simulink model "compositeload"  (R2023b)
settings: Solver=ode23t  StartTime=0.0  StopTime=30  RelTol=1e-2
libraries: spsThreePhaseDynamicLoadLib x3, spsAsynchronousMachinepuUnitsLib x3, spsThreePhaseVIMeasurementLib x3, spsThreePhaseSeriesRLCLoadLib x2, spsPower3phPhasorLib x1, spsThreePhasePISectionLineLib x1, spsThreePhaseTransformerTwoWindingsLib x1, spsThreePhaseBreakerLib x1, spsThreePhaseFaultLib x1, spsThreePhaseSourceLib x1, sps_lib x1
settings Model: Creator=Md. Kibria Saroare  LastModifiedBy=Md. Kibria Saroare

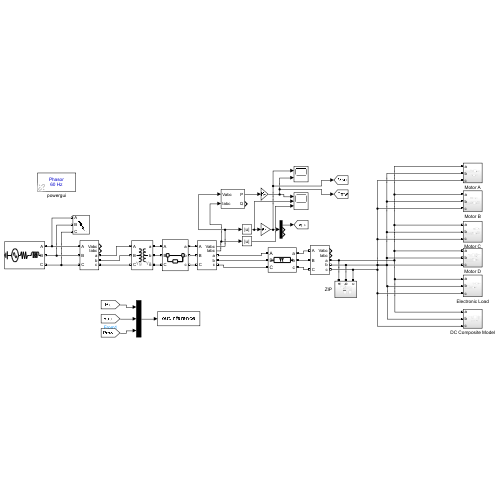
[thumbnail: Simulink's stored preview of the top-level diagram]
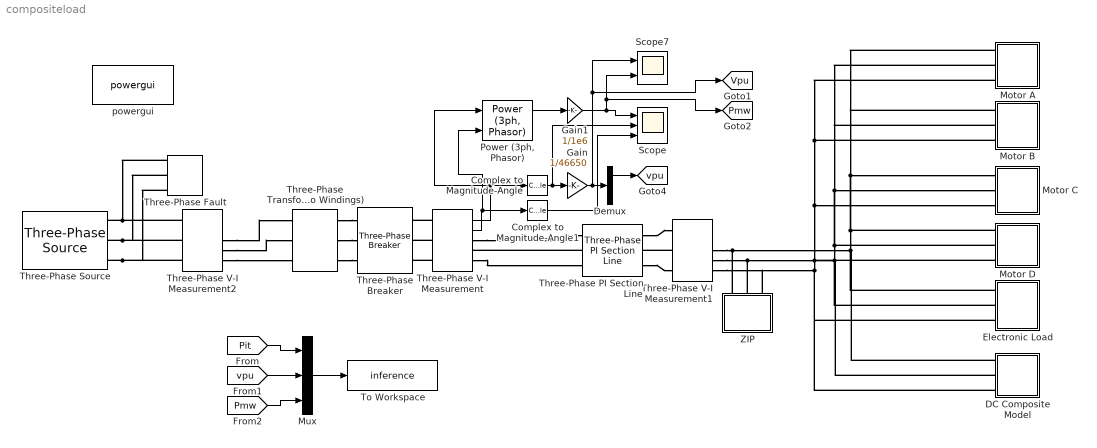
== system compositeload ==
  Complex to Magnitude-Angle : ComplexToMagnitudeAngle  Output=Magnitude
  Complex to Magnitude-Angle1 : ComplexToMagnitudeAngle  Output=Magnitude
  DC Composite Model : Subsystem
  Demux : Demux  Outputs=3
  Electronic Load : Subsystem
  Gain : Gain  Gain=1/46650
  Gain1 : Gain  Gain=1/1e6
  Motor A : Subsystem
  Motor B : Subsystem
  Motor C : Subsystem
  Motor D : Subsystem
  Mux : Mux  Inputs=3
  "Power (3ph, Phasor)" : spsPower3phPhasorLib/Power (3ph, Phasor)
      settings: LibrarySourceBlock=|
      | sps_lib/Sensors and Measurements/Power
      | (3ph, Phasor)
  Scope : Scope  NumInputPorts=3
  Scope7 : Scope  NumInputPorts=2
  Three-Phase PI Section Line : spsThreePhasePISectionLineLib/Three-Phase PI Section Line  LConnTagsString=a|b|c  RConnTagsString=A|B|C  Length=1  Frequency=60  Resistances=[ 0.3485 1.0455]  Inductances="[ 9.243e-4  2.773e-3]"  Capacitances=[1e-6 1e-6]
  Three-Phase Transformer (Two Windings) : spsThreePhaseTransformerTwoWindingsLib/Three-Phase Transformer (Two Windings)  Winding1Connection=Yg  Winding2Connection=Yg  CoreType=Three single-phase transformers  SetSaturation=off  Hysteresis=off  DataFile='hysteresis'  SetInitialFlux=off  Measurements=None  UNITS=pu  NominalPower=[ 2000e6 , 60 ]  Winding1=[2.3e+05 0.005 0.04]  Winding2=[33000 0.005 0.04]  Rm=500  Lm=500  L0=0.5  Saturation=[0 0;0.00035329 0.13044;0.1472 0.16522]  InitialFluxes=[ 0.8 , -0.8 , 0.7 ]  BreakLoop=off  DiscreteSolver=Trapezoidal iterative  DataType=off  TransfoNumber=1
  Three-Phase V-I Measurement : spsThreePhaseVIMeasurementLib/Three-Phase V-I Measurement  VoltageMeasurement=phase-to-phase  SetLabelV=off  LabelV=Vabc  Vpu=off  VpuLL=off  CurrentMeasurement=yes  SetLabelI=off  LabelI=Iabc  Ipu=off  Pbase=100e6  Vbase=500e3  OutputType=Complex  PhasorSimulation=on  PSBequivalent=0
  Three-Phase V-I Measurement1 : spsThreePhaseVIMeasurementLib/Three-Phase V-I Measurement  VoltageMeasurement=phase-to-phase  SetLabelV=off  LabelV=Vabc  Vpu=off  VpuLL=off  CurrentMeasurement=yes  SetLabelI=off  LabelI=Iabc  Ipu=off  Pbase=100e6  Vbase=500e3  OutputType=Complex  PhasorSimulation=on  PSBequivalent=0
  Three-Phase V-I Measurement2 : spsThreePhaseVIMeasurementLib/Three-Phase V-I Measurement  VoltageMeasurement=phase-to-phase  SetLabelV=off  LabelV=Vabc  Vpu=off  VpuLL=off  CurrentMeasurement=yes  SetLabelI=off  LabelI=Iabc  Ipu=off  Pbase=100e6  Vbase=500e3  OutputType=Complex  PhasorSimulation=on  PSBequivalent=0
  Three-Phase Breaker : spsThreePhaseBreakerLib/Three-Phase Breaker  InitialState=closed  SwitchA=on  SwitchB=on  SwitchC=on  SwitchTimes="[1/60  5/60]"  External=off  BreakerResistance=0.0001  SnubberResistance=1e6  SnubberCapacitance=inf  Measurements=None
  Three-Phase Fault : spsThreePhaseFaultLib/Three-Phase Fault  InitialStates=0  FaultA=on  FaultB=on  FaultC=on  GroundFault=on  SwitchTimes="[4  4.6]"  External=off  SwitchStatus=NaN  FaultResistance=0.001  GroundResistance=0.01  SnubberResistance=1e6  SnubberCapacitance=inf  Measurements=None
  Three-Phase Source : spsThreePhaseSourceLib/Three-Phase Source  InternalConnection=Yg  VoltagePhases=off  Voltage=230e3  PhaseAngle=0  Voltage_phases=[25e3 25e3 25e3]/sqrt(3)  PhaseAngles_phases=[0 -120 +120]  Frequency=60  NonIdealSource=on  SpecifyImpedance=on  Resistance=0.8929  Inductance=16.58e-3  ShortCircuitLevel=20000e6  BaseVoltage=230e3  XRratio=10  BusType=swing  Pref=10e3  Qref=0  Prefabc=[10e3, 10e3, 10e3]  Qrefabc=[0, 0, 0]  Qmin=-inf  Qmax=inf
  To Workspace : ToWorkspace  VariableName=inference  SaveFormat=Timeseries  SampleTime=-1
  ZIP : Subsystem
  powergui : sps_lib/powergui  Priority=1  SimulationMode=Phasor  SampleTime=50e-6  frequency=60  Iterations=50  frequencyindice=60  Pbase=100e6  ErrMax=1e-4  UnitsV=kV  UnitsW=MW  buscounter=0  FunctionMessages=off  echomessages=off  EnableUseOfTLC=off  CurrentSourceSwitches=off  DisableSnubberDevices=off  DisableRonSwitches=off  DisableVfSwitches=off  DisplayEquations=off  AutomaticDiscreteSolvers=off  SolverType=Tustin/Backward Euler (TBE)  Interpol=off  ExternalGateDelay=off  methode=off  Ts=100  x0status=blocks  SPID=on  SwTol=0  HookPort=off  NonlinearTolerance=1e-4  nMaxIteration=100  ContinueOnMaxIteration=off  RestoreLinks=warning  ResistiveCurrentMeasurement=off  Frange=[0:2:500]  Ylog=off  Xlog=on  ShowGrid=off  save=off  variable=ZData  structure=0  ZoomFFT=off  StartTime=0.0  cycles=1  DisplayStyle=1  fundamental=60  FreqAxis=off  MaxFrequency=1000  frequencyindicesteady=1  RmsSteady=1  display=off
  tag scope: Pmw=global, Vpu=global, vpu=global
  wires:
  Three-Phase V-I Measurement/1 -> Complex to Magnitude-Angle/1, "Power (3ph, Phasor)"/1
  Complex to Magnitude-Angle/1 -> Scope/2, Gain/1
  Gain/1 -> [Vpu], Scope7/1, Demux/1
  Demux/1 -> [vpu]
  Three-Phase V-I Measurement/2 -> "Power (3ph, Phasor)"/2, Complex to Magnitude-Angle1/1
  Complex to Magnitude-Angle1/1 -> Scope/3
  "Power (3ph, Phasor)"/1 -> Gain1/1
  Gain1/1 -> [Pmw], Scope7/2, Scope/1
  [Pit] -> Mux/1
  [vpu] -> Mux/2
  [Pmw] -> Mux/3
  Mux/1 -> To Workspace/1
  connections:
  Three-Phase Source/RConn1 -- Three-Phase V-I Measurement2/LConn1 -- Three-Phase Fault/LConn1
  Three-Phase Source/RConn2 -- Three-Phase V-I Measurement2/LConn2 -- Three-Phase Fault/LConn2
  Three-Phase Source/RConn3 -- Three-Phase V-I Measurement2/LConn3 -- Three-Phase Fault/LConn3
  Three-Phase Transformer (Two Windings)/RConn2 -- Three-Phase Breaker/LConn2
  Three-Phase Transformer (Two Windings)/RConn1 -- Three-Phase Breaker/LConn1
  Three-Phase Transformer (Two Windings)/RConn3 -- Three-Phase Breaker/LConn3
  Three-Phase V-I Measurement/LConn2 -- Three-Phase Breaker/RConn2
  Three-Phase V-I Measurement/LConn1 -- Three-Phase Breaker/RConn1
  Three-Phase V-I Measurement/LConn3 -- Three-Phase Breaker/RConn3
  Three-Phase PI Section Line/LConn2 -- Three-Phase V-I Measurement/RConn2
  Three-Phase V-I Measurement/RConn1 -- Three-Phase PI Section Line/LConn1
  Three-Phase V-I Measurement/RConn3 -- Three-Phase PI Section Line/LConn3
  Three-Phase V-I Measurement1/LConn2 -- Three-Phase PI Section Line/RConn2
  Three-Phase PI Section Line/RConn1 -- Three-Phase V-I Measurement1/LConn1
  Three-Phase PI Section Line/RConn3 -- Three-Phase V-I Measurement1/LConn3
  ZIP/LConn1 -- DC Composite Model/LConn1 -- Electronic Load/LConn1 -- Motor D/LConn1 -- Motor A/LConn1 -- Motor B/LConn1 -- Motor C/LConn1 -- Three-Phase V-I Measurement1/RConn1
  Three-Phase V-I Measurement2/RConn1 -- Three-Phase Transformer (Two Windings)/LConn1
  Three-Phase V-I Measurement2/RConn2 -- Three-Phase Transformer (Two Windings)/LConn2
  Three-Phase V-I Measurement2/RConn3 -- Three-Phase Transformer (Two Windings)/LConn3
  Three-Phase V-I Measurement1/RConn2 -- DC Composite Model/LConn2 -- Electronic Load/LConn2 -- Motor D/LConn2 -- Motor A/LConn2 -- Motor B/LConn2 -- Motor C/LConn2 -- ZIP/LConn2
  Motor A/LConn3 -- DC Composite Model/LConn3 -- Electronic Load/LConn3 -- ZIP/LConn3 -- Three-Phase V-I Measurement1/RConn3 -- Motor D/LConn3 -- Motor C/LConn3 -- Motor B/LConn3

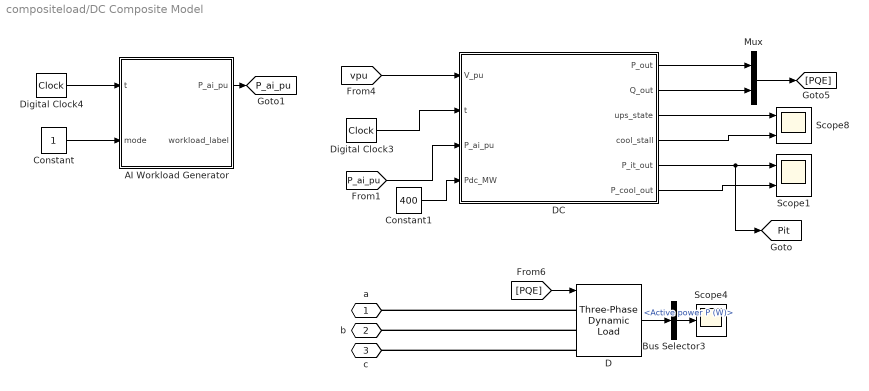
== system compositeload/DC Composite Model ==
  AI Workload Generator : MATLAB Function  TreatAsAtomicUnit=on  SystemSampleTime=0.001
  Bus Selector3 : BusSelector  OutputSignals=Active power P (W)
  Constant : Constant
  Constant1 : Constant  Value=400
  D : spsThreePhaseDynamicLoadLib/Three-Phase Dynamic Load  NominalVoltage=[ 33e3 60 ]  ActiveReactivePowers=[200e6 70e6]  PositiveSequence=[1 0]  ExternalControl=on  NpNq=[1.3 2]  TimeConstants="[0  0  0  0]"  MinimumVoltage=0.7  Tfilter=0.1  LoadFlowParameters=[4,0,0,0,0]
      settings: LibrarySourceBlock=|
      | sps_lib/Passives/Three-Phase
      | Dynamic Load
  DC : MATLAB Function  TreatAsAtomicUnit=on  SystemSampleTime=0.001
  Digital Clock3 : DigitalClock  SampleTime=0.001
  Digital Clock4 : DigitalClock  SampleTime=0.001
  Mux : Mux  Inputs=2
  Scope1 : Scope  NumInputPorts=2
  Scope4 : Scope
  Scope8 : Scope  NumInputPorts=2
  a : PMIOPort  Side=Left
  b : PMIOPort  Port=2  Side=Left
  c : PMIOPort  Port=3  Side=Left
  tag scope: P_ai_pu=global, Pit=global
  wires:
  D/1 -> Bus Selector3/1
  Bus Selector3/1 -> Scope4/1  "<Active power P (W)>"
  [PQE] -> D/1
  DC/4(cool_stall) -> Scope8/2
  DC/3(ups_state) -> Scope8/1
  DC/1(P_out) -> Mux/1
  Mux/1 -> [PQE]
  Digital Clock3/1 -> DC/2(t)
  [vpu] -> DC/1(V_pu)
  DC/2(Q_out) -> Mux/2
  DC/5(P_it_out) -> [Pit], Scope1/1
  DC/6(P_cool_out) -> Scope1/2
  Constant/1 -> AI Workload Generator/2(mode)
  Digital Clock4/1 -> AI Workload Generator/1(t)
  AI Workload Generator/1(P_ai_pu) -> [P_ai_pu]
  [P_ai_pu] -> DC/3(P_ai_pu)
  Constant1/1 -> DC/4(Pdc_MW)
  connections:
  D/LConn1 -- a/RConn1
  D/LConn3 -- c/RConn1
  D/LConn2 -- b/RConn1

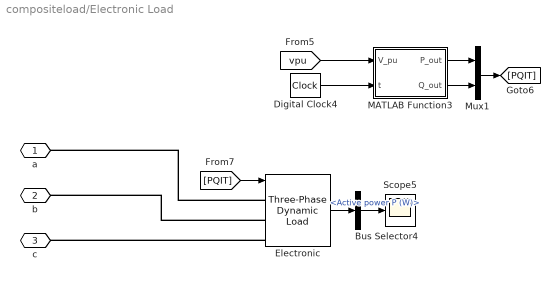
== system compositeload/Electronic Load ==
  Bus Selector4 : BusSelector  OutputSignals=Active power P (W)
  Digital Clock4 : DigitalClock  SampleTime=0.001
  Electronic : spsThreePhaseDynamicLoadLib/Three-Phase Dynamic Load  NominalVoltage=[ 33e3 60 ]  ActiveReactivePowers=[10.63e6 2.16e6]  PositiveSequence=[1 0]  ExternalControl=on  NpNq=[1.3 2]  TimeConstants="[0  0  0  0]"  MinimumVoltage=0.7  Tfilter=0.05  LoadFlowParameters=[4,0,0,0,0]
      settings: LibrarySourceBlock=|
      | sps_lib/Passives/Three-Phase
      | Dynamic Load
  MATLAB Function3 : MATLAB Function  TreatAsAtomicUnit=on  SystemSampleTime=0.001
  Mux1 : Mux  Inputs=2
  Scope5 : Scope
  a : PMIOPort  Side=Left
  b : PMIOPort  Port=2  Side=Left
  c : PMIOPort  Port=3  Side=Left
  wires:
  Electronic/1 -> Bus Selector4/1
  [PQIT] -> Electronic/1
  Bus Selector4/1 -> Scope5/1  "<Active power P (W)>"
  [vpu] -> MATLAB Function3/1(V_pu)
  MATLAB Function3/1(P_out) -> Mux1/1
  Digital Clock4/1 -> MATLAB Function3/2(t)
  Mux1/1 -> [PQIT]
  MATLAB Function3/2(Q_out) -> Mux1/2
  connections:
  Electronic/LConn3 -- c/RConn1
  Electronic/LConn2 -- b/RConn1
  Electronic/LConn1 -- a/RConn1

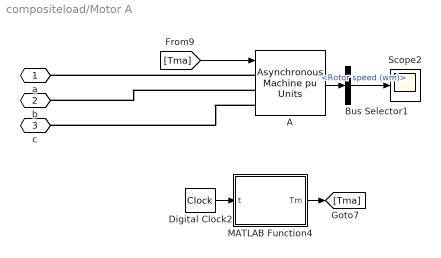
== system compositeload/Motor A ==
  A : spsAsynchronousMachinepuUnitsLib/Asynchronous Machine pu Units  RotorType=Squirrel-cage  PresetModel=No  MechanicalLoad=Torque Tm  ShowDetailedParameters=on  ReferenceFrame=Rotor  Units=pu  MeasurementBus=off  NominalParameters=[17.2e6 33e3 60]  VoltageRatio=1  Stator=[0.04 0.04]  Rotor=[0.0515 0.0839]  Cage1=[0.01909 0.0397]  Cage2=[0.01909 0.0397]  Lm=1.76  Mechanical=[0.5 0 2]  PolePairs=2  InitialConditions="[ 0.02,0   0,0,0   0,0,0 ]"  SimulateSaturation=off  Saturation="[0.212,0.4201,0.8125,1.0979,1.4799,2.2457,3.2586,4.5763,6.4763 ;   0.5,0.7,0.9,1,1.1,1.2 ,1.3,1.4,1.5]"  LoadFlowParameters=0  TsPowergui=0  TsBlock=-1  IterativeModel=Trapezoidal non iterative  IterativeDiscreteModel=Trapezoidal non iterative  Pmec=14.62e6
      settings: LibrarySourceBlock=|
      | sps_lib/Electrical Machines/Asynchronous Machine
      | pu Units
  Bus Selector1 : BusSelector  OutputSignals=Mechanical.Rotor speed (wm)
  Digital Clock2 : DigitalClock  SampleTime=0.001
  MATLAB Function4 : MATLAB Function  TreatAsAtomicUnit=on  SystemSampleTime=0.001
  Scope2 : Scope
  a : PMIOPort  Side=Left
  b : PMIOPort  Port=2  Side=Left
  c : PMIOPort  Port=3  Side=Left
  wires:
  A/1 -> Bus Selector1/1
  [Tma] -> A/1
  Bus Selector1/1 -> Scope2/1  "<Rotor speed (wm)>"
  MATLAB Function4/1(Tm) -> [Tma]
  Digital Clock2/1 -> MATLAB Function4/1(t)
  connections:
  A/LConn1 -- a/RConn1
  A/LConn2 -- b/RConn1
  A/LConn3 -- c/RConn1

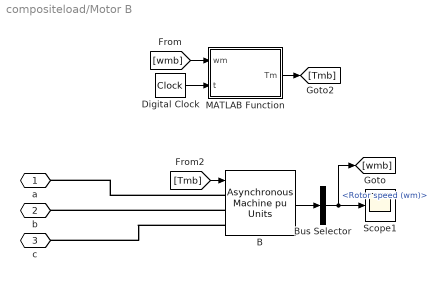
== system compositeload/Motor B ==
  B : spsAsynchronousMachinepuUnitsLib/Asynchronous Machine pu Units  RotorType=Squirrel-cage  PresetModel=No  MechanicalLoad=Torque Tm  ShowDetailedParameters=on  ReferenceFrame=Rotor  Units=pu  MeasurementBus=off  NominalParameters=[17.3e6 33e3 60]  VoltageRatio=1  Stator=[0.03 0.14]  Rotor=[0.0227 0.0516]  Cage1=[0.01909 0.0397]  Cage2=[0.01909 0.0397]  Lm=1.66  Mechanical=[0.5 0 2]  PolePairs=2  InitialConditions="[ 0.01,0   0,0,0   0,0,0 ]"  SimulateSaturation=off  Saturation="[0.212,0.4201,0.8125,1.0979,1.4799,2.2457,3.2586,4.5763,6.4763 ;   0.5,0.7,0.9,1,1.1,1.2 ,1.3,1.4,1.5]"  LoadFlowParameters=0  TsPowergui=0  TsBlock=-1  IterativeModel=Trapezoidal non iterative  IterativeDiscreteModel=Trapezoidal non iterative  Pmec=14.72e6
      settings: LibrarySourceBlock=|
      | sps_lib/Electrical Machines/Asynchronous Machine
      | pu Units
  Bus Selector : BusSelector  OutputSignals=Mechanical.Rotor speed (wm)
  Digital Clock : DigitalClock  SampleTime=0.001
  MATLAB Function : MATLAB Function  TreatAsAtomicUnit=on  SystemSampleTime=0.001
  Scope1 : Scope
  a : PMIOPort  Side=Left
  b : PMIOPort  Port=2  Side=Left
  c : PMIOPort  Port=3  Side=Left
  wires:
  [Tmb] -> B/1
  B/1 -> Bus Selector/1
  Bus Selector/1 -> [wmb], Scope1/1  "<Rotor speed (wm)>"
  MATLAB Function/1(Tm) -> [Tmb]
  [wmb] -> MATLAB Function/1(wm)
  Digital Clock/1 -> MATLAB Function/2(t)
  connections:
  B/LConn2 -- b/RConn1
  B/LConn3 -- c/RConn1
  B/LConn1 -- a/RConn1

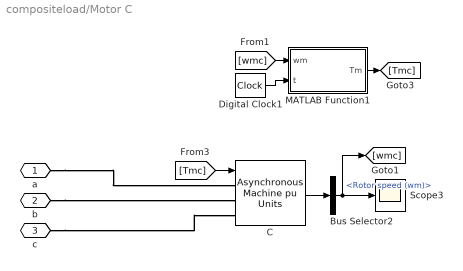
== system compositeload/Motor C ==
  Bus Selector2 : BusSelector  OutputSignals=Mechanical.Rotor speed (wm)
  C : spsAsynchronousMachinepuUnitsLib/Asynchronous Machine pu Units  RotorType=Squirrel-cage  PresetModel=No  MechanicalLoad=Torque Tm  ShowDetailedParameters=on  ReferenceFrame=Rotor  Units=pu  MeasurementBus=off  NominalParameters=[4.3e6 33e3 60]  VoltageRatio=1  Stator=[0.03 0.14]  Rotor=[0.0227 0.0516]  Cage1=[0.01909 0.0397]  Cage2=[0.01909 0.0397]  Lm=1.66  Mechanical=[0.1 0 2]  PolePairs=2  InitialConditions="[ 0.015,0   0,0,0   0,0,0 ]"  SimulateSaturation=off  Saturation="[0.212,0.4201,0.8125,1.0979,1.4799,2.2457,3.2586,4.5763,6.4763 ;   0.5,0.7,0.9,1,1.1,1.2 ,1.3,1.4,1.5]"  LoadFlowParameters=0  TsPowergui=0  TsBlock=-1  IterativeModel=Trapezoidal non iterative  IterativeDiscreteModel=Trapezoidal non iterative  Pmec=3.65e6
      settings: LibrarySourceBlock=|
      | sps_lib/Electrical Machines/Asynchronous Machine
      | pu Units
  Digital Clock1 : DigitalClock  SampleTime=0.001
  MATLAB Function1 : MATLAB Function  TreatAsAtomicUnit=on  SystemSampleTime=0.001
  Scope3 : Scope
  a : PMIOPort  Side=Left
  b : PMIOPort  Port=2  Side=Left
  c : PMIOPort  Port=3  Side=Left
  wires:
  C/1 -> Bus Selector2/1
  Bus Selector2/1 -> [wmc], Scope3/1  "<Rotor speed (wm)>"
  [Tmc] -> C/1
  [wmc] -> MATLAB Function1/1(wm)
  MATLAB Function1/1(Tm) -> [Tmc]
  Digital Clock1/1 -> MATLAB Function1/2(t)
  connections:
  a/RConn1 -- C/LConn1
  c/RConn1 -- C/LConn3
  b/RConn1 -- C/LConn2

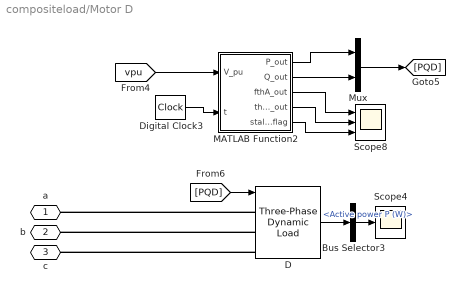
== system compositeload/Motor D ==
  Bus Selector3 : BusSelector  OutputSignals=Active power P (W)
  D : spsThreePhaseDynamicLoadLib/Three-Phase Dynamic Load  NominalVoltage=[ 33e3 60 ]  ActiveReactivePowers=[36.7e6 7.45e6]  PositiveSequence=[1 0]  ExternalControl=on  NpNq=[1.3 2]  TimeConstants="[0  0  0  0]"  MinimumVoltage=0.7  Tfilter=0.05  LoadFlowParameters=[4,0,0,0,0]
      settings: LibrarySourceBlock=|
      | sps_lib/Passives/Three-Phase
      | Dynamic Load
  Digital Clock3 : DigitalClock  SampleTime=0.001
  MATLAB Function2 : MATLAB Function  TreatAsAtomicUnit=on  SystemSampleTime=0.001
  Mux : Mux  Inputs=2
  Scope4 : Scope
  Scope8 : Scope  NumInputPorts=3
  a : PMIOPort  Side=Left
  b : PMIOPort  Port=2  Side=Left
  c : PMIOPort  Port=3  Side=Left
  wires:
  D/1 -> Bus Selector3/1
  Bus Selector3/1 -> Scope4/1  "<Active power P (W)>"
  [PQD] -> D/1
  MATLAB Function2/4(thetaA_out) -> Scope8/2
  MATLAB Function2/3(fthA_out) -> Scope8/1
  MATLAB Function2/1(P_out) -> Mux/1
  Mux/1 -> [PQD]
  MATLAB Function2/5(stall_flag) -> Scope8/3
  Digital Clock3/1 -> MATLAB Function2/2(t)
  [vpu] -> MATLAB Function2/1(V_pu)
  MATLAB Function2/2(Q_out) -> Mux/2
  connections:
  D/LConn1 -- a/RConn1
  D/LConn3 -- c/RConn1
  D/LConn2 -- b/RConn1

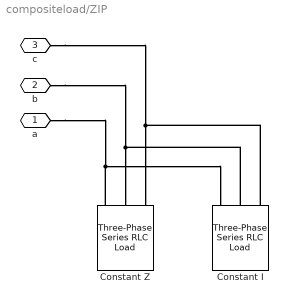
== system compositeload/ZIP ==
  Constant I : spsThreePhaseSeriesRLCLoadLib/Three-Phase Series RLC Load  LConnTagsString=A|B|C  Configuration=Y (grounded)  NominalVoltage=33e6  Vabc=[1e3 1e3 1e3]  Vabcp=[1e3 1e3 1e3]  NominalFrequency=60  UnbalancedPower=off  ActivePower=8.72e6  InductivePower=0  CapacitivePower=0.59e6  Pabc=[10e3 9e3 11e3]  QLabc=[100 90 110]  QCabc=[100 90 110]  Pabcp=[10e3 9e3 11e3]  QLabcp=[100 90 110]  QCabcp=[100 90 110]  Measurements=None  LoadType=constant I
  Constant Z : spsThreePhaseSeriesRLCLoadLib/Three-Phase Series RLC Load  LConnTagsString=A|B|C  Configuration=Y (grounded)  NominalVoltage=33e6  Vabc=[1e3 1e3 1e3]  Vabcp=[1e3 1e3 1e3]  NominalFrequency=60  UnbalancedPower=off  ActivePower=10.96e6  InductivePower=0  CapacitivePower=0.743e6  Pabc=[10e3 9e3 11e3]  QLabc=[100 90 110]  QCabc=[100 90 110]  Pabcp=[10e3 9e3 11e3]  QLabcp=[100 90 110]  QCabcp=[100 90 110]  Measurements=None  LoadType=constant Z
  a : PMIOPort  Side=Left
  b : PMIOPort  Port=2  Side=Left
  c : PMIOPort  Port=3  Side=Left
  connections:
  Constant I/LConn2 -- b/RConn1 -- Constant Z/LConn2
  Constant Z/LConn1 -- Constant I/LConn1 -- a/RConn1
  Constant I/LConn3 -- c/RConn1 -- Constant Z/LConn3

== matlab function compositeload/Motor C/MATLAB Function1 ==
  data: wm input; Tm output; t input
function Tm = motorC_torque(wm, t)
    wm_rated = 0.985;
    if t < 2.0
        ramp = t / 2.0;
    else
        ramp = 1.0;
    end
    Tm = ramp * (wm / wm_rated) * (wm / wm_rated);
end

== matlab function compositeload/Motor B/MATLAB Function ==
  data: wm input; Tm output; t input
function Tm = motorB_torque(wm, t)
    wm_rated = 0.99;
    if t < 2.0
        ramp = t / 2.0;
    else
        ramp = 1.0;
    end
    Tm = ramp * (wm / wm_rated) * (wm / wm_rated);
end

== matlab function compositeload/Motor D/MATLAB Function2 ==
  data: V_pu input; P_out output; Q_out output; t input; fthA_out output; thetaA_out output; stall_flag output
function [P_out, Q_out, fthA_out, thetaA_out, stall_flag] = motorD_phasor(V_pu, t)
%#codegen
% =========================================================================
% WECC Motor D: Single-Phase A/C Performance-Based Model (Final Version)
% =========================================================================
% Motor A portion (1-Frst = 80%): cannot restart after stalling
% Motor B portion (Frst = 20%): can restart after stalling
% Protection: thermal relay, contactor (hysteresis), UV relay (one-shot)
%
% Inputs:  V_pu  = per-unit voltage magnitude at load bus (scalar)
%          t     = simulation time (from Clock block)
% Outputs: P_out = active power in watts
%          Q_out = reactive power in vars
%          fthA_out   = fraction of Motor A not tripped by thermal relay
%          thetaA_out = internal temperature of Motor A
%          stall_flag = 1 if Motor A is stalled, 0 otherwise
%
% Block settings: sample time = 0.001 s
% =========================================================================

dt = 0.001;

% ===== SYSTEM PARAMETERS =====
Fmd   = 0.37;
Pload = 100e6;

% ===== MOTOR D PARAMETERS (Table 3 from paper) =====
CompPF = 0.98;      % power factor
Rstall = 0.1;       % stall resistance (pu)
Xstall = 0.1;       % stall reactance (pu)
Tstall = 0.033;     % stall time delay (s) - tuned slightly above 0.03
Frst   = 0.2;       % fraction that can restart
Vrst   = 0.95;      % restart voltage (pu)
Trst   = 0.3;       % restart time delay (s)
Fuvr_prot = 0.1;    % UV relay trip fraction
Vtr1   = 0.6;       % UV trip level 1 (pu)
Ttr1   = 0.02;      % UV trip delay 1 (s)
Vc1off = 0.5;       % contactor trip start (pu)
Vc2off = 0.4;       % contactor trip complete (pu)
Vc1on  = 0.6;       % contactor reconnect complete (pu)
Vc2on  = 0.5;       % contactor reconnect start (pu)
TTH    = 20;         % thermal time constant (s)
th1    = 1.4;        % thermal trip start temperature (pu)
th2    = 2.2;        % thermal trip complete temperature (pu)

% ===== DERIVED CONSTANTS =====
Zstall_sq = Rstall * Rstall + Xstall * Xstall;   % 0.02
Gstall    = Rstall / Zstall_sq;                    % 5.0
Bstall    = Xstall / Zstall_sq;                    % 5.0
P0        = 1.0;
Q0_prime  = tan(acos(CompPF)) - 6.0 * 0.14 * 0.14; % tan(acos(0.98)) - 6*(1-0.86)^2
Fbus      = 1.0;    % nominal frequency (pu)

% ===== PERSISTENT STATE VARIABLES =====
persistent stall_cntA stall_cntB rst_cnt
persistent is_stalledA is_stalledB
persistent thetaA thetaB fthA fthB
persistent fcon is_con_tripped
persistent fuvr uv1_tripped uv_cnt1
persistent init_done

if isempty(init_done)
    stall_cntA    = 0;
    stall_cntB    = 0;
    rst_cnt       = 0;
    is_stalledA   = false;
    is_stalledB   = false;
    thetaA        = 0;
    thetaB        = 0;
    fthA          = 1.0;
    fthB          = 1.0;
    fcon          = 1.0;
    is_con_tripped = false;
    fuvr          = 1.0;
    uv1_tripped   = false;
    uv_cnt1       = 0;
    init_done     = true;
end

% ===== SOFT START (network settling) =====
if t < 0.5
    P_out      = Fmd * Pload;
    Q_out      = Fmd * Pload * tan(acos(CompPF));
    fthA_out   = 1.0;
    thetaA_out = 0.0;
    stall_flag = 0.0;
    return;
end

% ===== INPUT CONDITIONING =====
V = double(V_pu(1));
if V < 0.01
    V = 0.01;
end
if V > 1.5
    V = 1.5;
end

% ===== FIND V'stall (intersection point) =====
Vstall_prime = 0.6;
for Vt = 0.40:0.005:0.65
    pst    = Gstall * Vt * Vt;
    p_comp = P0 + 12.0 * power(0.86 - Vt, 3.2);
    if p_comp < pst
        Vstall_prime = Vt;
        break;
    end
end

% =========================================================================
% P-V AND Q-V PERFORMANCE CURVES (Paper Section 3.3.2)
% Region 1: V > 0.8         -> normal running
% Region 2: V'stall <= V <= 0.8  -> transition (approaching stall)
% Region 3: V < V'stall     -> stall impedance (Gstall*V^2, -Bstall*V^2)
% =========================================================================

if V > 0.8
    P_run = P0 * (1.0 + (1.0 - Fbus));
    Q_run = Q0_prime + 6.0 * (V - 0.86) * (V - 0.86) * (1.0 - 3.3 * (1.0 - Fbus));
elseif V >= Vstall_prime
    P_run = P0 + 12.0 * power(0.86 - V, 3.2) * (1.0 + (1.0 - Fbus));
    Q_run = Q0_prime + 11.0 * power(0.86 - V, 2.5) * (1.0 - 3.3 * (1.0 - Fbus));
else
    P_run = P0;
    Q_run = Q0_prime;
end

P_stall = Gstall * V * V;
Q_stall = -Bstall * V * V;

% =========================================================================
% STALLING LOGIC
% Motor A (1-Frst = 80%): stalls permanently, tripped only by thermal relay
% Motor B (Frst = 20%): stalls but can restart if V > Vrst for Trst seconds
% =========================================================================

% ----- Motor A: cannot restart -----
if ~is_stalledA
    if V < Vstall_prime
        stall_cntA = stall_cntA + dt;
        if stall_cntA >= Tstall
            is_stalledA = true;
            stall_cntA = 0;
        end
    else
        stall_cntA = 0;
    end
end

% ----- Motor B: can restart -----
if ~is_stalledB
    if V < Vstall_prime
        stall_cntB = stall_cntB + dt;
        if stall_cntB >= Tstall
            is_stalledB = true;
            stall_cntB = 0;
        end
    else
        stall_cntB = 0;
    end
else
    if V >= Vrst
        rst_cnt = rst_cnt + dt;
        if rst_cnt >= Trst
            is_stalledB = false;
            rst_cnt = 0;
            thetaB = 0;
        end
    else
        rst_cnt = 0;
    end
end

% =========================================================================
% THERMAL RELAY (Paper Figure 6)
% theta = filtered I^2*R through first-order lag with time constant TTH
% fth = 1           if theta < th1
% fth = 1-(theta-th1)/(th2-th1)  if th1 <= theta < th2
% fth = 0           if theta >= th2
% =========================================================================

% ----- Motor A thermal -----
if is_stalledA
    I_sq = V * V / Zstall_sq;
    heat_in = I_sq * Rstall;
    thetaA = thetaA + (heat_in - thetaA) / TTH * dt;
    if thetaA < 0
        thetaA = 0;
    end
    if thetaA >= th2
        fthA = 0;
    elseif thetaA >= th1
        fthA = 1.0 - (thetaA - th1) / (th2 - th1);
        if fthA < 0
            fthA = 0;
        end
    else
        fthA = 1.0;
    end
else
    if thetaA > 0.001
        thetaA = thetaA * (1.0 - dt / TTH);
    else
        thetaA = 0;
    end
    fthA = 1.0;
end

% ----- Motor B thermal -----
if is_stalledB
    I_sq = V * V / Zstall_sq;
    heat_in = I_sq * Rstall;
    thetaB = thetaB + (heat_in - thetaB) / TTH * dt;
    if thetaB < 0
        thetaB = 0;
    end
    if thetaB >= th2
        fthB = 0;
    elseif thetaB >= th1
        fthB = 1.0 - (thetaB - th1) / (th2 - th1);
        if fthB < 0
            fthB = 0;
        end
    else
        fthB = 1.0;
    end
else
    if thetaB > 0.001
        thetaB = thetaB * (1.0 - dt / TTH);
    else
        thetaB = 0;
    end
    fthB = 1.0;
end

% =========================================================================
% CONTACTOR MODEL (Paper Figure 7 — hysteresis)
% Trip path:      V decreasing -> trips between Vc1off and Vc2off
% Reconnect path: V increasing -> reconnects between Vc2on and Vc1on
% =========================================================================

if ~is_con_tripped
    if V <= Vc2off
        fcon = 0;
        is_con_tripped = true;
    elseif V < Vc1off
        fcon = (V - Vc2off) / (Vc1off - Vc2off);
    else
        fcon = 1.0;
    end
else
    if V >= Vc1on
        fcon = 1.0;
        is_con_tripped = false;
    elseif V >= Vc2on
        fcon = (V - Vc2on) / (Vc1on - Vc2on);
    else
        fcon = 0;
    end
end

% =========================================================================
% UV RELAY (Paper Section — one-shot per level, permanent trip)
% Level 1: V < Vtr1 for Ttr1 seconds -> trip Fuvr_prot fraction (once)
% Level 2: Ttr2 = 9999 -> effectively disabled
% =========================================================================

if ~uv1_tripped
    if V < Vtr1
        uv_cnt1 = uv_cnt1 + dt;
        if uv_cnt1 >= Ttr1
            fuvr = 1.0 - Fuvr_prot;
            uv1_tripped = true;
        end
    else
        uv_cnt1 = 0;
    end
end

% =========================================================================
% OUTPUT: COMBINE MOTOR A + MOTOR B
% =========================================================================

if is_stalledA
    PA = P_stall * fthA;
    QA = Q_stall * fthA;
else
    PA = P_run;
    QA = Q_run;
end

if is_stalledB
    PB = P_stall * fthB;
    QB = Q_stall * fthB;
else
    PB = P_run;
    QB = Q_run;
end

P_pu = (1.0 - Frst) * PA + Frst * PB;
Q_pu = (1.0 - Frst) * QA + Frst * QB;

% Apply protection
P_pu = P_pu * fcon * fuvr;
Q_pu = Q_pu * fcon * fuvr;

if P_pu < 0
    P_pu = 0;
end

% Scale to physical units
P_out = P_pu * Fmd * Pload;
Q_out = Q_pu * Fmd * Pload;

% Diagnostic outputs
fthA_out   = fthA;
thetaA_out = thetaA;
if is_stalledA
    stall_flag = 1.0;
else
    stall_flag = 0.0;
end

end

== matlab function compositeload/Electronic Load/MATLAB Function3 ==
  data: V_pu input; P_out output; Q_out output; t input
function [P_out, Q_out] = electronic_load(V_pu, t)
%#codegen
Fel   = 0.106286;
Pload = 100e6;
PFel  = 0.98;
Vd1   = 0.7;
Vd2   = 0.5;
frcel = 1.0;

Pel0 = Fel * Pload;
Qel0 = Pel0 * tan(acos(PFel));

% Soft start
if t < 0.5
    P_out = Pel0;
    Q_out = Qel0;
    return;
end

persistent Vmin_track init_done

if isempty(init_done)
    Vmin_track = 1.0;
    init_done = true;
end

% Force scalar and protect
V = double(V_pu(1));
if V < 0.01
    V = 0.01;
end
if V > 1.5
    V = 1.5;
end

% Track minimum voltage
% KEY FIX: Only track Vmin while voltage is DECREASING
% Once voltage starts recovering, Vmin stays at the lowest point reached
if V < Vmin_track
    Vmin_track = V;
end

% Clamp Vmin to Vd2 floor
if Vmin_track < Vd2
    Vmin_track = Vd2;
end

% Compute voltage-dependent load fraction
if Vmin_track <= Vd2
    % Voltage went below Vd2: all load tripped
    % But can partially recover based on frcel
    if V >= Vd1
        Fvl = frcel;  % partial recovery above Vd1
    elseif V > Vd2
        Fvl = frcel * (V - Vd2) / (Vd1 - Vd2);
    else
        Fvl = 0;
    end
elseif V < Vd1
    if V <= Vmin_track
        % Voltage still decreasing
        Fvl = (V - Vd2) / (Vd1 - Vd2);
    else
        % Voltage recovering above Vmin
        base = (Vmin_track - Vd2) / (Vd1 - Vd2);
        recovery = frcel * (V - Vmin_track) / (Vd1 - Vd2);
        Fvl = base + recovery;
    end
else
    % V >= Vd1
    if Vmin_track >= Vd1
        % Voltage never went below Vd1
        Fvl = 1.0;
    else
        % Voltage recovered above Vd1 after dipping
        base = (Vmin_track - Vd2) / (Vd1 - Vd2);
        recovery = frcel * (V - Vmin_track) / (Vd1 - Vd2);
        Fvl = base + recovery;
    end
end

% Clamp between 0 and 1
if Fvl < 0
    Fvl = 0;
end
if Fvl > 1.0
    Fvl = 1.0;
end

P_out = Fvl * Pel0;
Q_out = Fvl * Qel0;

end

== matlab function compositeload/Motor A/MATLAB Function4 ==
  data: Tm output; t input
% In a MATLAB Function block for Motor A torque
function Tm = motorA_ramp(t)
    if t < 2.0
        Tm = t / 2.0;    % ramp from 0 to 1 pu over 2 seconds
    else
        Tm = 1.0;
    end
end

== matlab function compositeload/DC Composite Model/AI Workload Generator ==
  data: t input; mode input; P_ai_pu output; workload_label output
function [P_ai_pu, workload_label] = ai_workload(t, mode)
%#codegen
% AI GPU Workload Profile Generator
% mode: 1=Training, 2=Inference, 3=Idle
% Output: P_ai_pu (0 to 1), workload_label

workload_label = double(mode);

if mode == 1
    % TRAINING: sustained high with checkpoint dips
    base_power = 0.3;
    checkpoint_interval = 60.0;
    checkpoint_duration = 2.0;
    checkpoint_dip = 0.40;
    comm_period = 1.2;
    comm_amplitude = 0.6;
    
    time_in_cycle = mod(t, checkpoint_interval);
    if time_in_cycle < checkpoint_duration
        P_ai_pu = checkpoint_dip;
    else
        oscillation = comm_amplitude * sin(2.0 * 3.14159 * t / comm_period);
        P_ai_pu = base_power + oscillation;
    end
    
elseif mode == 2
    % INFERENCE: bursty multi-frequency
    base_power = 0.15;
    burst1 = 0.25 * sin(2.0 * 3.14159 * t / 5.0);
    burst2 = 0.15 * sin(2.0 * 3.14159 * t / 1.3);
    burst3 = 0.10 * sin(2.0 * 3.14159 * t / 0.4);
    
    if t < 2.0
        diurnal = 0.5 + 0.5 * (t / 2.0);
    else
        diurnal = 1.0;
    end
    
    P_ai_pu = (base_power + burst1 + burst2 + burst3) * diurnal;
    
elseif mode == 3
    % IDLE
    P_ai_pu = 0.15;
else
    P_ai_pu = 0.5;
end

if P_ai_pu < 0.05
    P_ai_pu = 0.05;
end
if P_ai_pu > 1.0
    P_ai_pu = 1.0;
end

end

== matlab function compositeload/DC Composite Model/DC ==
  data: V_pu input; P_out output; Q_out output; t input; ups_state output; cool_stall output; P_it_out output; P_ai_pu input; P_cool_out output; Pdc_MW input
function [P_out, Q_out, ups_state, cool_stall, P_it_out, P_cool_out] = ...
    datacenter_motorE(V_pu, t, P_ai_pu, Pdc_MW)
%#codegen
% =========================================================================
% WECC CLM Extension: Data Center Load Model (Motor E)
% Scalable from 100 MW to 500 MW
% =========================================================================
% Inputs:  V_pu    = per-unit voltage at load bus
%          t       = simulation time
%          P_ai_pu = AI workload demand (0-1 pu)
%          Pdc_MW  = data center rated power in MW (100 to 500)
%
% Outputs: P_out (W), Q_out (VAR)
%          ups_state, cool_stall, P_it_out, P_cool_out
%
% Block sample time = 0.001
% =========================================================================

dt = 0.001;

% ===== DATA CENTER SIZING =====
Pdc = double(Pdc_MW(1)) * 1e6;    % convert MW to W

% ===== SUB-COMPONENT FRACTIONS =====
% Based on industry data:
% IT load (servers/GPUs): 55-65% -> 60%
% Cooling (chillers/CRAH): 25-35% -> 30%
% Auxiliary (lighting/office/network): 8-12% -> 10%
Fit_max  = 0.60;
Fcool    = 0.30;
Faux     = 0.10;

% ===== UPS PARAMETERS =====
% Large DC UPS: tighter voltage tolerance, faster transfer
V_ups_trip    = 0.90;    % static transfer switch threshold
V_ups_return  = 0.95;    % return to grid threshold
T_ups_battery = 30.0;    % battery hold-up time (s)
T_diesel_start = 12.0;   % diesel generator start time (s)
T_ups_transfer = 0.004;  % static switch transfer time (s)
PF_it = 0.95;

% ===== COOLING PARAMETERS =====
% Industrial chillers: higher inertia, different stall characteristics
Rstall_c = 0.10;     Xstall_c = 0.12;
Vstall_c = 0.55;     % industrial compressors stall lower than residential
Tstall_c = 0.05;     % stall confirmation delay
Vrst_c   = 0.90;     Trst_c = 2.0;   % slower restart (large chillers)
TTH_c    = 60;        % higher thermal mass (industrial)
th1_c    = 1.6;       th2_c = 2.8;    % wider thermal margin
PF_cool  = 0.85;

% ===== VFD COOLING FRACTION =====
% Modern DCs use VFDs on some chillers (don't stall, ride through)
Fvfd = 0.40;    % 40% of cooling on VFDs (constant power during fault)

% ===== PERSISTENT STATE =====
persistent ups_mode batt_timer diesel_timer transfer_cnt
persistent is_cool_stalled cool_stall_cnt cool_rst_cnt
persistent theta_cool fth_cool
persistent P_it_before_fault
persistent rebound_active rebound_timer
persistent init_done

if isempty(init_done)
    ups_mode          = 0;
    batt_timer        = 0;
    diesel_timer      = 0;
    transfer_cnt      = 0;
    is_cool_stalled   = false;
    cool_stall_cnt    = 0;
    cool_rst_cnt      = 0;
    theta_cool        = 0;
    fth_cool          = 1;
    P_it_before_fault = 0;
    rebound_active    = false;
    rebound_timer     = 0;
    init_done         = true;
end

% Soft start
if t < 1.0
    ramp = t / 1.0;
    P_out = Pdc * 0.7 * ramp;
    Q_out = Pdc * 0.25 * ramp;
    ups_state  = 0;
    cool_stall = 0;
    P_it_out   = Fit_max * Pdc * 0.9 * ramp;
    P_cool_out = Fcool * Pdc * ramp;
    return;
end

V = double(V_pu(1));
if V < 0.01
    V = 0.01;
end
if V > 1.5
    V = 1.5;
end

P_ai = double(P_ai_pu(1));
if P_ai < 0.05
    P_ai = 0.05;
end
if P_ai > 1.0
    P_ai = 1.0;
end

% =========================================================
% COMPONENT 1: IT LOAD WITH UPS + AI WORKLOAD
% =========================================================
P_it_demand = Fit_max * Pdc * P_ai;
Q_it_demand = P_it_demand * tan(acos(PF_it));

P_it = 0;
Q_it = 0;

if ups_mode == 0
    % GRID-CONNECTED: IT load on grid, scaled by workload
    P_it_before_fault = P_it_demand;
    
    if V < V_ups_trip
        ups_mode = 1;
        batt_timer = 0;
        diesel_timer = 0;
        transfer_cnt = 0;
    end
    
    P_it = P_it_demand;
    Q_it = Q_it_demand;
    
elseif ups_mode == 1
    % UPS BATTERY MODE: IT load invisible to grid
    batt_timer = batt_timer + dt;
    diesel_timer = diesel_timer + dt;
    transfer_cnt = transfer_cnt + dt;
    
    if transfer_cnt < T_ups_transfer
        % During transfer: partial load visible
        P_it = P_it_before_fault * 0.3;
        Q_it = Q_it_demand * 0.3;
    else
        % Fully on battery: zero grid draw
        P_it = 0;
        Q_it = 0;
    end
    
    if V >= V_ups_return
        % Voltage recovered: LOAD REBOUND
        ups_mode = 0;
        rebound_active = true;
        rebound_timer = 0;
        batt_timer = 0;
    elseif diesel_timer >= T_diesel_start
        ups_mode = 2;
    elseif batt_timer >= T_ups_battery
        ups_mode = 0;  % forced return
        rebound_active = true;
        rebound_timer = 0;
    end
    
elseif ups_mode == 2
    % DIESEL BACKUP: permanently off grid
    P_it = 0;
    Q_it = 0;
end

% LOAD REBOUND: IT load returns to grid with inrush
% Causes a secondary voltage dip
if rebound_active
    rebound_timer = rebound_timer + dt;
    rebound_duration = 0.5;  % 500ms rebound transient
    
    if rebound_timer < rebound_duration
        % During rebound: 120% of pre-fault load (inrush)
        rebound_factor = 1.2 - 0.2 * (rebound_timer / rebound_duration);
        P_it = P_it * rebound_factor;
        Q_it = Q_it * rebound_factor * 1.5;  % higher Q during rebound
    else
        rebound_active = false;
    end
end

% =========================================================
% COMPONENT 2: COOLING LOAD (split: motor + VFD)
% =========================================================

Zstall_sq = Rstall_c * Rstall_c + Xstall_c * Xstall_c;
Gstall_cool = Rstall_c / Zstall_sq;
Bstall_cool = Xstall_c / Zstall_sq;

% Cooling demand proportional to IT workload
cool_scale = 0.6 + 0.4 * P_ai;  % 60-100% cooling

P_cool_base = Fcool * Pdc * cool_scale;
Q_cool_base = P_cool_base * tan(acos(PF_cool));

% --- Motor-driven portion (1-Fvfd): can stall ---
P_motor_rated = (1.0 - Fvfd) * P_cool_base;
Q_motor_rated = (1.0 - Fvfd) * Q_cool_base;

P_motor_stall = Gstall_cool * V * V * (1.0 - Fvfd) * Fcool * Pdc;
Q_motor_stall = -Bstall_cool * V * V * (1.0 - Fvfd) * Fcool * Pdc;

% Stall logic (motor portion only)
if ~is_cool_stalled
    if V < Vstall_c
        cool_stall_cnt = cool_stall_cnt + dt;
        if cool_stall_cnt >= Tstall_c
            is_cool_stalled = true;
            cool_stall_cnt = 0;
        end
    else
        cool_stall_cnt = 0;
    end
else
    if V >= Vrst_c
        cool_rst_cnt = cool_rst_cnt + dt;
        if cool_rst_cnt >= Trst_c
            is_cool_stalled = false;
            cool_rst_cnt = 0;
            theta_cool = 0;
        end
    else
        cool_rst_cnt = 0;
    end
end

% Thermal relay
if is_cool_stalled
    I_sq = V * V / Zstall_sq;
    theta_cool = theta_cool + (I_sq * Rstall_c - theta_cool) / TTH_c * dt;
    if theta_cool < 0
        theta_cool = 0;
    end
    if theta_cool >= th2_c
        fth_cool = 0;
    elseif theta_cool >= th1_c
        fth_cool = 1.0 - (theta_cool - th1_c) / (th2_c - th1_c);
        if fth_cool < 0
            fth_cool = 0;
        end
    else
        fth_cool = 1.0;
    end
else
    if theta_cool > 0.001
        theta_cool = theta_cool * (1.0 - dt / TTH_c);
    else
        theta_cool = 0;
    end
    fth_cool = 1.0;
end

% Motor cooling output
if is_cool_stalled
    P_motor = P_motor_stall * fth_cool;
    Q_motor = Q_motor_stall * fth_cool;
else
    P_motor = P_motor_rated * V * V;
    Q_motor = Q_motor_rated * V * V;
end

% --- VFD portion (Fvfd): rides through, constant power ---
% VFDs maintain constant power down to ~0.5 pu voltage
if V >= 0.5
    P_vfd = Fvfd * P_cool_base;
    Q_vfd = Fvfd * Q_cool_base * 0.5;  % VFDs have lower Q
elseif V >= 0.3
    % Linear reduction below 0.5
    vfd_frac = (V - 0.3) / 0.2;
    P_vfd = Fvfd * P_cool_base * vfd_frac;
    Q_vfd = Fvfd * Q_cool_base * 0.5 * vfd_frac;
else
    P_vfd = 0;
    Q_vfd = 0;
end

P_cool = P_motor + P_vfd;
Q_cool = Q_motor + Q_vfd;

% =========================================================
% COMPONENT 3: AUXILIARY (constant impedance)
% =========================================================
P_aux = Faux * Pdc * V * V;
Q_aux = Faux * Pdc * 0.15 * V * V;

% =========================================================
% TOTAL DATA CENTER OUTPUT
% =========================================================
P_out = P_it + P_cool + P_aux;
Q_out = Q_it + Q_cool + Q_aux;

if P_out < 0
    P_out = 0;
end

ups_state = double(ups_mode);
if is_cool_stalled
    cool_stall = 1.0;
else
    cool_stall = 0.0;
end
P_it_out = P_it;
P_cool_out = P_cool;

end
